simulink model "modelRubBeRAdvanced"  (R2024b)
settings: Solver=ode4  StartTime=0.0  StopTime=inf  FixedStep=settings.samplingTime_s  MaxStep=1e-2  RelTol=1e-5
PostLoadFcn:
  | , if any(exist('dsrtsu_mdlpostloadfcn', 'file') == [2, 3, 6]), try dsrtsu_mdlpostloadfcn('Execute', bdroot); catch fprintf('Error in PostLoadFcn (dsrtsu_mdlpostloadfcn) for model "%s":\n %s\n', bdroot, lasterr); end, end,
  | , if any(exist('dsrtsu_mdlpostloadfcn', 'file') ~= 0), dsrtsu_mdlpostloadfcn('Execute', bdroot); end,
values from neighbouring files (symbols this model uses):
  virtualRubber =     [virtualRubBeR.mat]
libraries: simulink x1
Description:
  | Standard RTI1202 template.
  | Supported MATLAB version:  R2019b.
settings Model: Tag=RTI1202  DSRTSU_INTERNAL_RTI_VER=490  DSRTSU_INTERNAL_RTI_TYPE=rti1202  RTICANMMDATA=struct('GeneralSetupData',struct('modelroot','C:\UNI\Master\04_MA\05_Experiments','generalsettings',struct('filesettings',struct('destfolder',struct('Name','RTICANMM_FILES','Check',1),'buildfolder',struct('Name','.','Check',1),'AbsDestfolder',struct('Name','C:\UNI\Master\04_MA\05_Experiments\RTICANMM_FILES'),'AbsBuildfolder',struct('Name','C:\UNI\Master\04_MA\05_Experiments'))),'options',struct('addpaths',1,'rmpaths',1,'addtrcexclusion',true,'cannavigator',struct('checkmonitoring',0),'show_usrtrc',0,'use_usrtrc',0),'advanced',struct('options',ones(1,100)),'MPSetup',{{}},'RTI',struct('Type','RTI1202','Ver','7.13','Date','02-Nov-2019'),'modelname','PLL_autoStep_r2019b_rti','block','PLL_autoStep_r2019b_rti'))  DSRTSU_INTERNAL_RTIFPGA=80  Creator=patri  LastModifiedBy=phippold
settings SolverCC: AlgebraicLoopSolver=TrustRegion
settings DataIOCC: ReturnWorkspaceOutputs=off
settings OptimizationCC: BlockReduction=off  OptimizeBlockIOStorage=off  BufferReuse=off  GlobalBufferReuse=off  ExpressionFolding=off  LocalBlockOutputs=off
settings DebuggingCC: UnconnectedInputMsg=warning  UnconnectedOutputMsg=warning  UnconnectedLineMsg=warning  ArithmeticOperatorsInVariantConditions=warning
settings HardwareCC: TargetIntDivRoundTo=Zero  TargetEndianess=BigEndian  TargetHWDeviceType=Custom Processor->Custom
settings ModelReferenceCC: EnableRefExpFcnMdlSchedulingChecks=on
settings SFSimCC: SimUseLocalCustomCode=off  CustomCodeUndefinedFunction=UseInterfaceOnly
settings RTWCC: RTWUseLocalCustomCode=off  GPUComputeCapability=3.5  DLArmComputeVersion=19.05
settings CodeAppCC: StateflowObjectComments=on
settings ConfigComp: CovMetricSettings=dswe
settings SimscapeCC: SimscapeNormalizeSystem=off

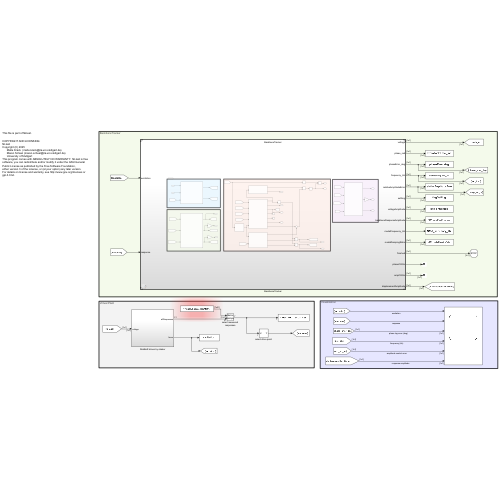
[thumbnail: Simulink's stored preview of the top-level diagram]
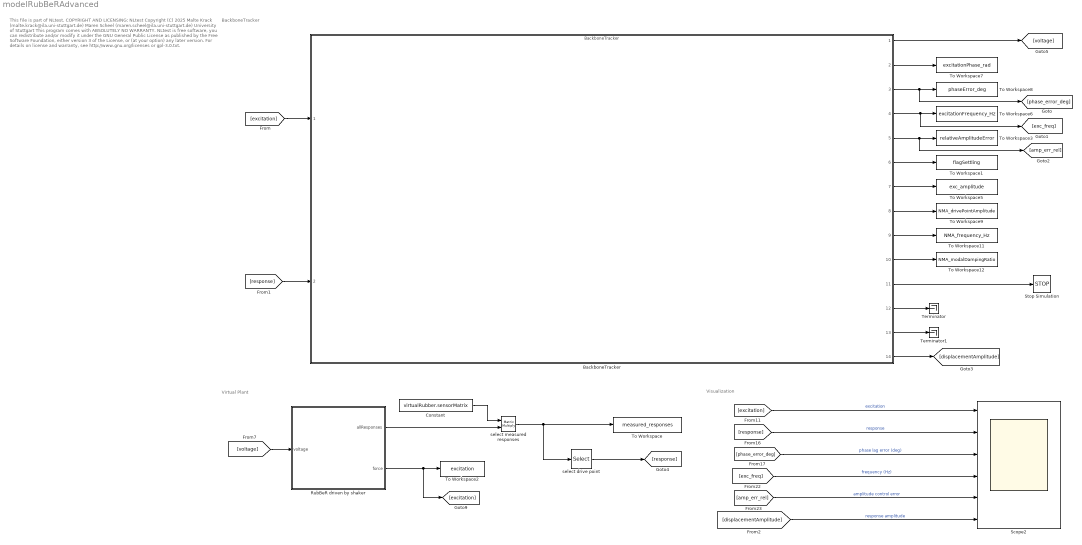
== system modelRubBeRAdvanced ==
  note: BackboneTracker
  note: Visualization
  note: Virtual Plant
  note: This file is part of NLtest.
      |
      | COPYRIGHT AND LICENSING:
      | NLtest
      | Copyright (C) 2025
      | Malte Krack (malte.krack@ila.uni-stuttgart.de)
      | Maren Scheel (maren.scheel@ila.uni-stuttgart.de)
      | University of Stuttgart
      | This program comes with ABSOLUTELY NO WARRANTY. NLtest is free software, you can redistribute and/or modify it under the GNU General Public License as published by the Free Software Foundation,
      | either version 3 of the License, or (at your option) any later version.
      | For details on license and warranty, see http://www.gnu.org/licenses or gpl-3.0.txt.
  BackboneTracker : ModelReference  ModelNameDialog=BackboneTracker.slx  SimulationMode=Normal  ModelReferenceVersion=17.4
  Constant : Constant  Value=virtualRubber.sensorMatrix
  RubBeR driven by shaker : Subsystem
  Scope2 : Scope  NumInputPorts=6
  Stop Simulation : Stop
  Terminator : Terminator
  Terminator1 : Terminator
  To Workspace : ToWorkspace  VariableName=measured_responses  SaveFormat=Structure With Time  SampleTime=-1
  To Workspace1 : ToWorkspace  VariableName=flagSettling  SaveFormat=Structure With Time  SampleTime=-1
  To Workspace11 : ToWorkspace  VariableName=NMA_frequency_Hz  SaveFormat=Structure With Time  SampleTime=-1
  To Workspace12 : ToWorkspace  VariableName=NMA_modalDampingRatio  SaveFormat=Structure With Time  SampleTime=-1
  To Workspace2 : ToWorkspace  VariableName=excitation  SaveFormat=Structure With Time  SampleTime=-1
  To Workspace3 : ToWorkspace  VariableName=relativeAmplitudeError  SaveFormat=Structure With Time  SampleTime=-1
  To Workspace5 : ToWorkspace  VariableName=exc_amplitude  SaveFormat=Structure With Time  SampleTime=-1
  To Workspace6 : ToWorkspace  VariableName=excitationFrequency_Hz  SaveFormat=Structure With Time  SampleTime=-1
  To Workspace7 : ToWorkspace  VariableName=excitationPhase_rad  SaveFormat=Structure With Time  SampleTime=-1
  To Workspace8 : ToWorkspace  VariableName=phaseError_deg  SaveFormat=Structure With Time  SampleTime=-1
  To Workspace9 : ToWorkspace  VariableName=NMA_drivePointAmplitude  SaveFormat=Structure With Time  SampleTime=-1
  select drive point : Selector  IndexOptions=Index vector (dialog)  Indices=settings.indexSensorDrivePoint  OutputSizes=1
  select measured responses : Product  Multiplication=Matrix(*)
  wires:
  select measured responses/1 -> select drive point/1, To Workspace/1
  [voltage] -> RubBeR driven by shaker/1(voltage)
  RubBeR driven by shaker/2(force) -> [excitation], To Workspace2/1
  [excitation] -> Scope2/1  "excitation"
  [response] -> Scope2/2  "response"
  [phase_error_deg] -> Scope2/3  "phase lag error (deg)"
  [exc_freq] -> Scope2/4  "frequency (Hz)"
  [amp_err_rel] -> Scope2/5  "amplitude control error"
  [displacementAmplitude] -> Scope2/6  "response amplitude"
  select drive point/1 -> [response]
  BackboneTracker/2 -> To Workspace7/1
  BackboneTracker/3 -> [phase_error_deg], To Workspace8/1
  BackboneTracker/5 -> [amp_err_rel], To Workspace3/1
  BackboneTracker/4 -> [exc_freq], To Workspace6/1
  BackboneTracker/6 -> To Workspace1/1
  BackboneTracker/7 -> To Workspace5/1
  BackboneTracker/10 -> To Workspace12/1
  BackboneTracker/9 -> To Workspace11/1
  BackboneTracker/8 -> To Workspace9/1
  BackboneTracker/11 -> Stop Simulation/1
  BackboneTracker/12 -> Terminator/1
  BackboneTracker/13 -> Terminator1/1
  BackboneTracker/1 -> [voltage]
  [excitation] -> BackboneTracker/1
  [response] -> BackboneTracker/2
  RubBeR driven by shaker/1(allResponses) -> select measured responses/2
  Constant/1 -> select measured responses/1
  BackboneTracker/14 -> [displacementAmplitude]

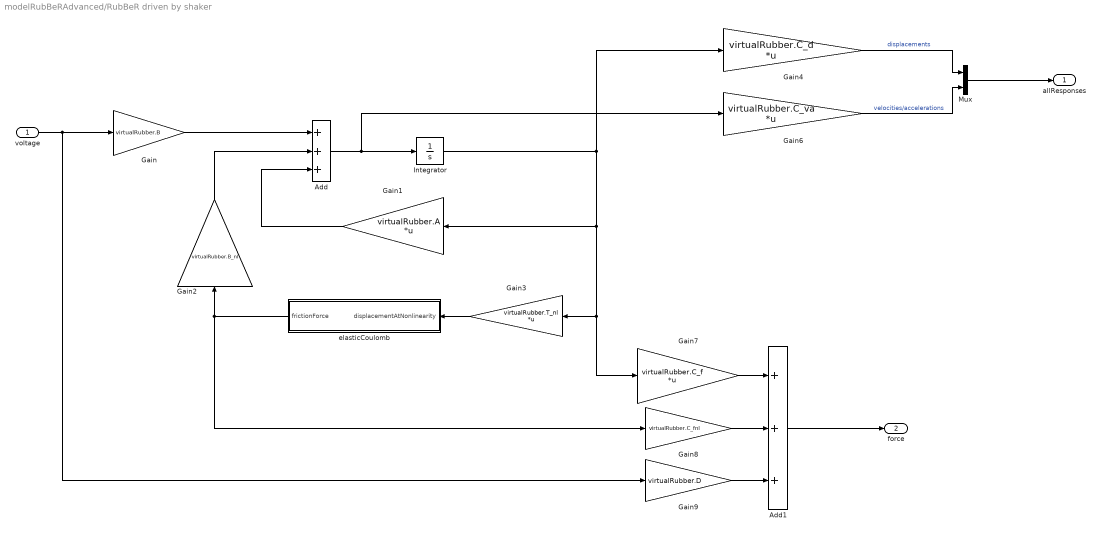
== system modelRubBeRAdvanced/RubBeR driven by shaker ==
  voltage : Inport
  Add : Sum  Inputs=+++
  Add1 : Sum  Inputs=+++
  Gain : Gain  Gain=virtualRubber.B
  Gain1 : Gain  Gain=virtualRubber.A  Multiplication=Matrix(K*u) (u vector)
  Gain2 : Gain  Gain=virtualRubber.B_nl
  Gain3 : Gain  Gain=virtualRubber.T_nl  Multiplication=Matrix(K*u)
  Gain4 : Gain  Gain=virtualRubber.C_d  Multiplication=Matrix(K*u) (u vector)
  Gain6 : Gain  Gain=virtualRubber.C_va  Multiplication=Matrix(K*u) (u vector)
  Gain7 : Gain  Gain=virtualRubber.C_f  Multiplication=Matrix(K*u) (u vector)
  Gain8 : Gain  Gain=virtualRubber.C_fnl
  Gain9 : Gain  Gain=virtualRubber.D
  Integrator : Integrator
  Mux : Mux  Inputs=2
  elasticCoulomb : Subsystem
  allResponses : Outport
  force : Outport  Port=2
  wires:
  voltage/1 -> Gain9/1, Gain/1
  Gain/1 -> Add/1
  Add/1 -> Integrator/1, Gain6/1
  Gain1/1 -> Add/3
  Gain2/1 -> Add/2
  elasticCoulomb/1(frictionForce) -> Gain2/1, Gain8/1
  Gain3/1 -> elasticCoulomb/1(displacementAtNonlinearity)
  Integrator/1 -> Gain4/1, Gain1/1, Gain3/1, Gain7/1
  Gain7/1 -> Add1/1
  Gain8/1 -> Add1/2
  Gain9/1 -> Add1/3
  Add1/1 -> force/1
  Gain4/1 -> Mux/1  "displacements"
  Gain6/1 -> Mux/2  "velocities/accelerations"
  Mux/1 -> allResponses/1

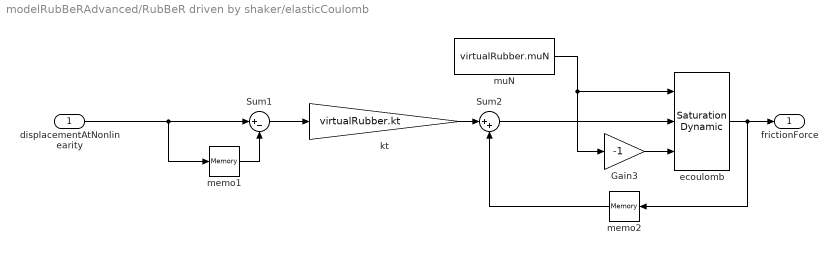
== system modelRubBeRAdvanced/RubBeR driven by shaker/elasticCoulomb ==
  displacementAtNonlinearity : Inport
  Gain3 : Gain  Gain=-1
  Sum1 : Sum  Inputs=|+-
  Sum2 : Sum  Inputs=|++
  ecoulomb : simulink/Discontinuities/Saturation Dynamic  OutMin=[]  OutMax=[]  OutDataTypeStr=Inherit: Same as second input  OutDataType=fixdt(1, 16)  OutScaling=2^-10  DoSatur=off
  kt : Gain  Gain=virtualRubber.kt
  memo1 : Memory
  memo2 : Memory
  muN : Constant  Value=virtualRubber.muN
  frictionForce : Outport
  wires:
  Sum1/1 -> kt/1
  kt/1 -> Sum2/1
  muN/1 -> ecoulomb/1, Gain3/1
  Gain3/1 -> ecoulomb/3
  Sum2/1 -> ecoulomb/2
  ecoulomb/1 -> frictionForce/1, memo2/1
  memo2/1 -> Sum2/2
  displacementAtNonlinearity/1 -> Sum1/1, memo1/1
  memo1/1 -> Sum1/2
